simulink model "TestModelv1"  (R2021b)
settings: Solver=VariableStepAuto  StartTime=0.0  StopTime=20  RelTol=1e-3
values from neighbouring files (symbols this model uses):
  a = 0.3    [TestModelv1_init.m]
  b = 0.8    [TestModelv1_init.m]
  g = 9.81    [TestModelv1_init.m]
  h = 0.3    [TestModelv1_init.m]
  k2 = (b*g)/(V*V*sin(lambda)-b*g*cos(lambda))    [TestModelv1_init.m]
  V = 1.46    [TestModelv1_init.m]
settings Model: Creator=Raj Shah  LastModifiedBy=Raj Shah

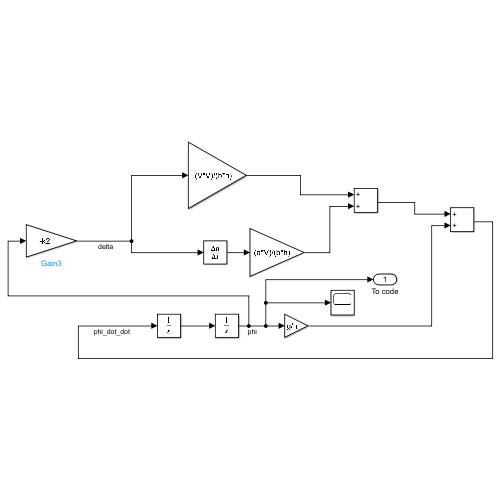
[thumbnail: Simulink's stored preview of the top-level diagram]
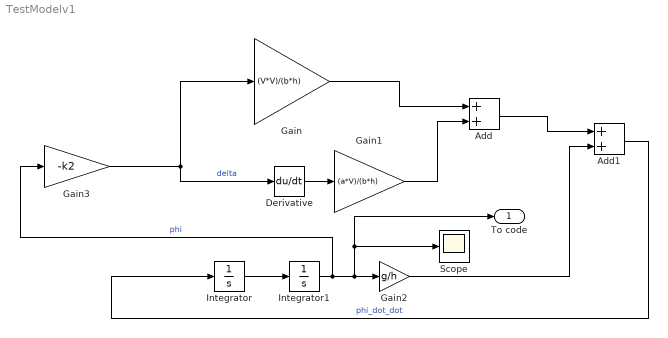
== system TestModelv1 ==
  Add : Sum
  Add1 : Sum
  Derivative : Derivative
  Gain : Gain  Gain=(V*V)/(b*h)
  Gain1 : Gain  Gain=(a*V)/(b*h)
  Gain2 : Gain  Gain=g/h
  Gain3 : Gain  Gain=-k2
  Integrator : Integrator
  Integrator1 : Integrator  InitialCondition=0.17453
  Scope : Scope
  To code : Outport
  wires:
  Derivative/1 -> Gain1/1
  Gain1/1 -> Add/2
  Gain/1 -> Add/1
  Integrator/1 -> Integrator1/1
  Add1/1 -> Integrator/1  "phi_dot_dot"
  Integrator1/1 -> Gain3/1, Scope/1, To code/1, Gain2/1  "phi"
  Add/1 -> Add1/1
  Gain2/1 -> Add1/2
  Gain3/1 -> Derivative/1, Gain/1  "delta"
